simulink model "PipeModel_detailed"  (R2020a)
settings: Solver=ode3  StartTime=0.0  StopTime=10000  FixedStep=dt  RelTol=1e-3
settings Model: Creator=saif  LastModifiedBy=Afraz
settings DataIOCC: LimitDataPoints=on  SaveFormat=Array  ReturnWorkspaceOutputs=off
settings OptimizationCC: BlockReduction=off  BooleanDataType=off  LifeSpan=inf
settings DebuggingCC: SaveWithParameterizedLinksMsg=none  UnderspecifiedInitializationDetection=Classic  MergeDetectMultiDrivingBlocksExec=none  SignalResolutionControl=TryResolveAllWithWarning  SFUnexpectedBacktrackingDiag=warning  SFNoUnconditionalDefaultTransitionDiag=warning  ArithmeticOperatorsInVariantConditions=warning
settings HardwareCC: ProdBitPerPointer=32  ProdBitPerSizeT=32  ProdBitPerPtrDiffT=32  ProdLargestAtomicFloat=None  ProdIntDivRoundTo=Undefined  ProdEndianess=Unspecified  ProdWordSize=32  ProdHWDeviceType=32-bit Generic  TargetUnknown=on
settings ModelReferenceCC: PropagateSignalLabelsOutOfModel=off
settings SFSimCC: SimUseLocalCustomCode=off  CustomCodeUndefinedFunction=UseInterfaceOnly
settings RTWCC: RTWUseLocalCustomCode=off
settings CodeAppCC: StateflowObjectComments=on
settings GRTTargetCC: TargetLangStandard=C89/C90 (ANSI)
settings ConfigComp: CovMetricSettings=dw  CovHtmlReporting=on  CovSaveCumulativeToWorkspaceVar=on  CovSaveSingleToWorkspaceVar=on  CovExternalEMLEnable=off  CovSFcnEnable=off

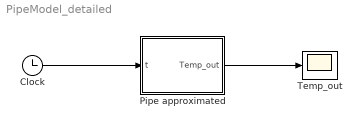
== system PipeModel_detailed ==
  Clock : Clock
  Pipe approximated : Subsystem
  Temp_out : Scope
  wires:
  Clock/1 -> Pipe approximated/1(t)
  Pipe approximated/1(Temp_out) -> Temp_out/1

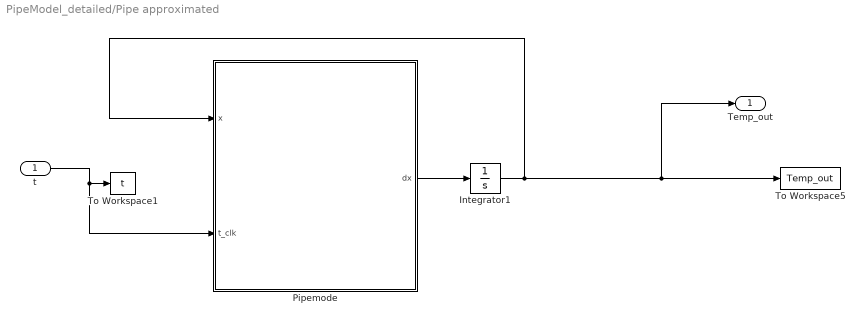
== system PipeModel_detailed/Pipe approximated ==
  t : Inport
  Integrator1 : Integrator  InitialCondition=273.15
  Pipemode : MATLAB Function  TreatAsAtomicUnit=on
  To Workspace1 : ToWorkspace  VariableName=t  SampleTime=-1
  To Workspace5 : ToWorkspace  VariableName=Temp_out  SampleTime=-1
  Temp_out : Outport
  wires:
  Pipemode/1(dx) -> Integrator1/1
  t/1 -> To Workspace1/1, Pipemode/2(t_clk)
  Integrator1/1 -> Temp_out/1, To Workspace5/1, Pipemode/1(x)

== matlab function PipeModel_detailed/Pipe approximated/Pipemode ==
  data: x input; t_clk input; dx output; param parameter
function dx  = fcn(x,t_clk, param)
%#codegen

%param=[rho cp L D_ins_out Tb K  D_pipe flowrate A v  R C ];
 dx = zeros(1,1);

 dx1= -(x-param(5))/(param(12)*param(11)); % dx1 is Temp in K
 dx = [dx1];
% Temp_out=Temp_out;
